simulink model "Yaw_Diff_SS_C"  (R2013a)
settings: Solver=ode45  StartTime=0.0  StopTime=30  RelTol=1e-3
values from neighbouring files (symbols this model uses):
  Drag = D    [State_Space_Yaw_C.m]
  K_Yaw_C = lqr(A,B,Q,R)    [State_Space_Yaw_C.m]
  omega_0 = 520    [State_Space_Yaw_C.m]    (also in State_Space_Yaw_D_2.m)
  YawStep = 1    [State_Space_Yaw_C.m]    (also in State_Space_Yaw_D_2.m)
undefined symbols (not defined in the file or in its folder): I_Psi, J, Kw, Motor_TimeConstant, Speed_yIntercept
libraries: simulink x2
settings Model: Creator=Ross  LastModifiedBy=Ross

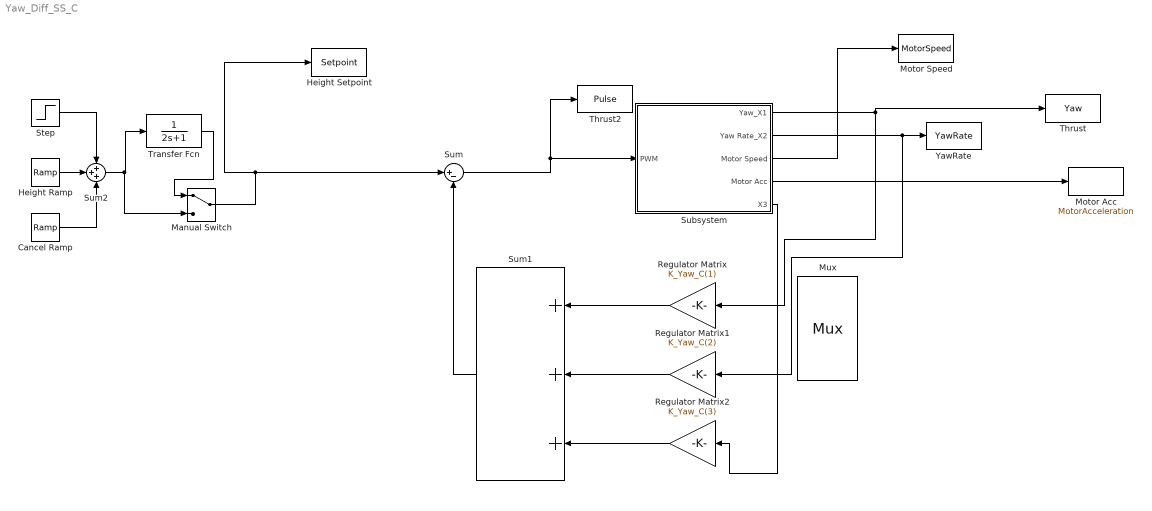
== system Yaw_Diff_SS_C ==
  Cancel Ramp : simulink/Sources/Ramp  slope=-1  start=5  X0=0
  Height Ramp : simulink/Sources/Ramp  slope=1  start=1  X0=0
  Height Setpoint : ToWorkspace  VariableName=Setpoint  SampleTime=-1  SaveFormat=Timeseries
  Manual Switch : ManualSwitch
  Motor Acc : ToWorkspace  VariableName=MotorAcceleration  SampleTime=-1  SaveFormat=Timeseries
  Motor Speed : ToWorkspace  VariableName=MotorSpeed  SampleTime=-1  SaveFormat=Timeseries
  Mux : Mux  Inputs=3
      settings: DisplayOption=signals
  Regulator Matrix : Gain  Gain=K_Yaw_C(1)
  Regulator Matrix1 : Gain  Gain=K_Yaw_C(2)
  Regulator Matrix2 : Gain  Gain=K_Yaw_C(3)
  Step : Step  Time=10  After=YawStep  SampleTime=0
  Subsystem : Subsystem
  Sum : Sum  Inputs=|+-
  Sum1 : Sum  Inputs=+++
  Sum2 : Sum  Inputs=+++
  Thrust : ToWorkspace  VariableName=Yaw  SampleTime=-1  SaveFormat=Timeseries
  Thrust2 : ToWorkspace  VariableName=Pulse  SampleTime=-1  SaveFormat=Timeseries
  Transfer Fcn : TransferFcn  Denominator=[2 1]
  YawRate : ToWorkspace  VariableName=YawRate  SampleTime=-1  SaveFormat=Timeseries
  wires:
  Step/1 -> Sum2/1
  Height Ramp/1 -> Sum2/2
  Cancel Ramp/1 -> Sum2/3
  Sum2/1 -> Manual Switch/2, Transfer Fcn/1
  Manual Switch/1 -> Height Setpoint/1, Sum/1
  Subsystem/1(Yaw_X1) -> Regulator Matrix/1, Thrust/1
  Subsystem/3(Motor Speed) -> Motor Speed/1
  Subsystem/2(Yaw Rate_X2) -> Regulator Matrix1/1, YawRate/1
  Subsystem/4(Motor Acc) -> Motor Acc/1
  Subsystem/5(X3) -> Regulator Matrix2/1
  Sum/1 -> Thrust2/1, Subsystem/1(PWM)
  Regulator Matrix/1 -> Sum1/1
  Regulator Matrix1/1 -> Sum1/2
  Regulator Matrix2/1 -> Sum1/3
  Sum1/1 -> Sum/2
  Transfer Fcn/1 -> Manual Switch/1

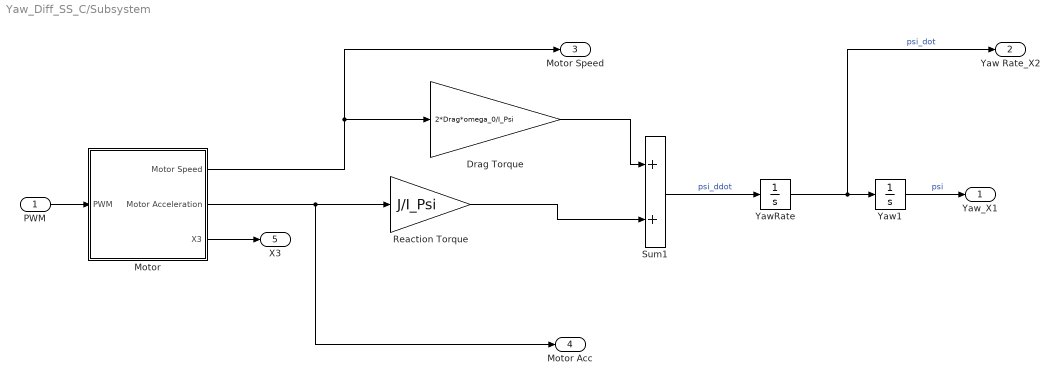
== system Yaw_Diff_SS_C/Subsystem ==
  PWM : Inport
  Drag Torque : Gain  Gain=2*Drag*omega_0/I_Psi
  Motor : Subsystem
  Reaction Torque : Gain  Gain=J/I_Psi
  Sum1 : Sum
  Yaw1 : Integrator  LowerSaturationLimit=0
  YawRate : Integrator
  Yaw_X1 : Outport
  Yaw Rate_X2 : Outport  Port=2
  Motor Speed : Outport  Port=3
  Motor Acc : Outport  Port=4
  X3 : Outport  Port=5
  wires:
  PWM/1 -> Motor/1(PWM)
  Motor/2(Motor Acceleration) -> Motor Acc/1, Reaction Torque/1
  Yaw1/1 -> Yaw_X1/1  "psi"
  YawRate/1 -> Yaw Rate_X2/1, Yaw1/1  "psi_dot"
  Sum1/1 -> YawRate/1  "psi_ddot"
  Drag Torque/1 -> Sum1/1
  Motor/1(Motor Speed) -> Drag Torque/1, Motor Speed/1
  Reaction Torque/1 -> Sum1/2
  Motor/3(X3) -> X3/1

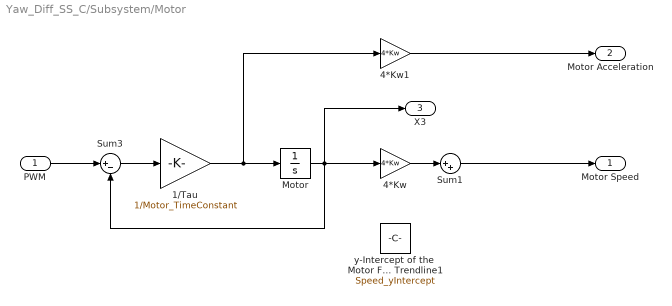
== system Yaw_Diff_SS_C/Subsystem/Motor ==
  PWM : Inport
  1/Tau : Gain  Gain=1/Motor_TimeConstant
  4*Kw : Gain  Gain=4*Kw
  4*Kw1 : Gain  Gain=4*Kw
  Motor : Integrator
  Sum1 : Sum  Inputs=|++
  Sum3 : Sum  Inputs=|+-
  y-Intercept of the  Motor Forc Trendline1 : Constant  Value=Speed_yIntercept
  Motor Speed : Outport
  Motor Acceleration : Outport  Port=2
  X3 : Outport  Port=3
  wires:
  1/Tau/1 -> 4*Kw1/1, Motor/1
  Motor/1 -> X3/1, 4*Kw/1, Sum3/2
  PWM/1 -> Sum3/1
  Sum3/1 -> 1/Tau/1
  4*Kw/1 -> Sum1/1
  Sum1/1 -> Motor Speed/1
  4*Kw1/1 -> Motor Acceleration/1
